simulink model "SlidesExample"  (Simulink 7.7)
settings: Solver=FixedStepDiscrete  StartTime=0.0  StopTime=120  FixedStep=0.5  MaxStep=1  RelTol=1e-3
undefined symbols (not defined in the file or in its folder): BLOM_FunctionCode, thetak, vk, xk, yk
libraries: MPCMdlLib x12
settings Model: Creator=vichik  LastModifiedBy=Frank
settings OptimizationCC: InitFltsAndDblsToZero=on
settings DebuggingCC: StrictBusMsg=Warning

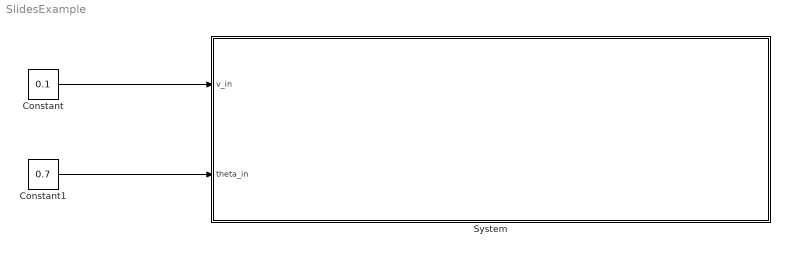
== system SlidesExample ==
  Constant : Constant  Value=0.1
  Constant1 : Constant  Value=0.7
  System : Subsystem
  wires:
  Constant/1 -> System/1(v_in)
  Constant1/1 -> System/2(theta_in)

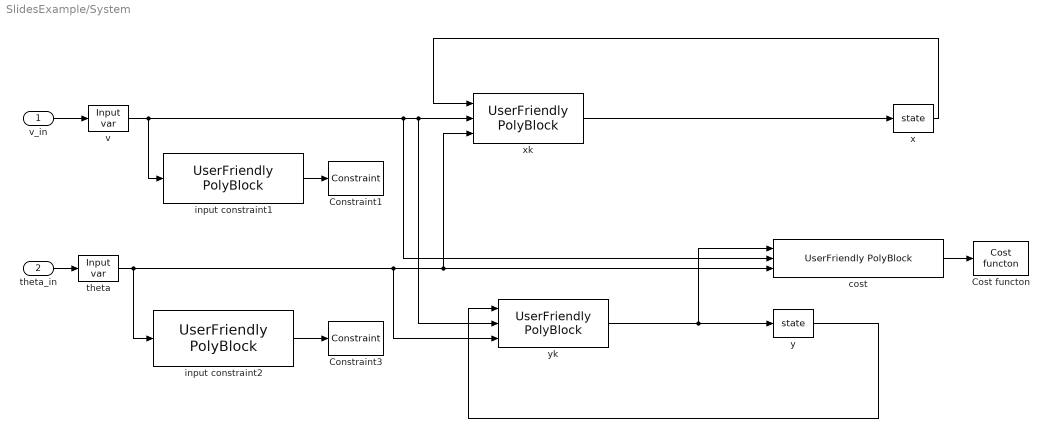
== system SlidesExample/System ==
  v_in : Inport
  theta_in : Inport  Port=2
  Constraint1 : MPCMdlLib/Constraint  Tag=InequalBlock  CompareSign=< 0
  Constraint3 : MPCMdlLib/Constraint  Tag=InequalBlock  CompareSign=< 0
  Cost functon : MPCMdlLib/Cost functon  Tag=OptCost
  "cost " : MPCMdlLib/UserFriendly PolyBlock  Tag=PolyBlock  A=[0 2 0; 0 0 2;2 0 0;1 0 0;0 0 0]  C=[1 1 1 -10 25]  gA=[0 0 0]  gC=1  input_type=Scalar  output_type=Scalar  port_names=yk,vk,thetak
  input constraint1 : MPCMdlLib/UserFriendly PolyBlock  Tag=PolyBlock  A="[1  ;  0 ]"  C=[1 -1 ; -1 0]  gA="[0  ]"  gC=1  input_type=Scalar  output_type=Vector  port_names=v
  input constraint2 : MPCMdlLib/UserFriendly PolyBlock  Tag=PolyBlock  A=[1;0]  C="[1 -pi/2; -1  0]"  gA=[0]  gC=1  input_type=Scalar  output_type=Vector  port_names=theta
  theta : MPCMdlLib/Input var  Tag=OptInput  SystemSampleTime=-1  step_ratio=1  save_name=BL_System_theta
  v : MPCMdlLib/Input var  Tag=OptInput  SystemSampleTime=-1  step_ratio=1  save_name=BL_System_v
  x : MPCMdlLib/state  Tag=OptState  SystemSampleTime=-1  init_val=0  save_name=BL_System_x
  xk : MPCMdlLib/UserFriendly PolyBlock  Tag=PolyBlock  A=[1 0 0;0 1 BLOM_FunctionCode('cos')]  C=[1 0.5]  gA=[0 0 0]  gC=1  input_type=Scalar  output_type=Scalar  port_names=xk,vk,thetak
  y : MPCMdlLib/state  Tag=OptState  SystemSampleTime=-1  init_val=y0  save_name=BL_System_y
  yk : MPCMdlLib/UserFriendly PolyBlock  Tag=PolyBlock  A=[1 0 0; 0 1 BLOM_FunctionCode('sin')]  C=[1 0.5]  gA=[0 0 0]  gC=1  input_type=Scalar  output_type=Scalar  port_names=yk,vk,thetak
  wires:
  xk/1 -> x/1
  x/1 -> xk/1
  v/1 -> "cost "/2, xk/2, yk/2, input constraint1/1
  "cost "/1 -> Cost functon/1
  v_in/1 -> v/1
  input constraint1/1 -> Constraint1/1
  theta_in/1 -> theta/1
  theta/1 -> input constraint2/1, yk/3, "cost "/3, xk/3
  yk/1 -> "cost "/1, y/1
  y/1 -> yk/1
  input constraint2/1 -> Constraint3/1
